simulink model "npc_controller"  (R2022a)
settings: Solver=FixedStepDiscrete  StartTime=0.0  StopTime=20  RelTol=1e-3  EnableMultiTasking=on
values from neighbouring files (symbols this model uses):
  Tsw = 1.5E-5    [param.sldd]
undefined symbols (not defined in the file or in its folder): CAN_O_INT, CANA_BASE, Down, GPTRIP1SEL, GPTRIP2SEL, GPTRIP3SEL, TZ1, TZ2, TZ3, Up
libraries: simulink x153, hdlsllib x90, c2802xlib x34, c2837xDlib x18, c280xlib x12, canmsglib x9, c2838xlib x8, idelinklib_common x3, c2806xlib x2, slpidlib x2, c28004xlib x2, c281xlib x2
(part 11 of 45)

== system npc_controller/CONTROL/SVPWM/SVPWM2/detSeq ==
  subsector : Inport  OutDataTypeStr=double  PortDimensions=1
  f : TriggerPort  TriggerType=function-call  VariantControl=(inherit)
      settings: CopyFcn=Stateflow.SLINSF.SimulinkMan.removeBlockPreDeleteFcn  PreDeleteFcn=Stateflow.SLINSF.SimulinkMan.unsafePredeleteFcn
  Cast To Double : DataTypeConversion  OutDataTypeStr=double  SaturateOnIntegerOverflow=off  RndMeth=Floor
  Cast To Double1 : DataTypeConversion  OutDataTypeStr=double  SaturateOnIntegerOverflow=off  RndMeth=Floor
  Cast To Double2 : DataTypeConversion  OutDataTypeStr=double  SaturateOnIntegerOverflow=off  RndMeth=Floor
  Constant{,5,7..8,12,17} (6 alike) : Constant  Value=[0 1 1 1]
  Constant1 : Constant  Value=[0 1 0 1]
  Constant{2..3,10..11,14..15} (6 alike) : Constant  Value=[0 0 0 1]
  Constant13 : Constant  Value=[0 1 0 1]
  Constant16 : Constant  Value=[0 0 1 1]
  Constant18 : Constant  Commented=on  Value=[1 1 0 0]
  Constant19 : Constant  Commented=on  Value=[1 0 0 0]
  Constant20 : Constant  Commented=on  Value=[1 1 1 0]
  Constant21 : Constant  Commented=on  Value=[1 1 1 0]
  Constant22 : Constant  Commented=on  Value=[1 1 0 0]
  Constant23 : Constant  Commented=on  Value=[1 0 0 0]
  Constant24 : Constant  Commented=on  Value=[1 0 0 0]
  Constant25 : Constant  Commented=on  Value=[1 1 1 0]
  Constant26 : Constant  Commented=on  Value=[1 1 0 0]
  Constant4 : Constant  Value=[0 0 1 1]
  Constant6 : Constant  Value=[0 0 1 1]
  Constant9 : Constant  Value=[0 1 0 1]
  Multiport Switch : MultiPortSwitch  Inputs=6  DataPortForDefault=Additional data port  SaturateOnIntegerOverflow=off  InputSameDT=off
  Multiport Switch1 : MultiPortSwitch  Inputs=6  DataPortForDefault=Additional data port  SaturateOnIntegerOverflow=off  InputSameDT=off
  Multiport Switch2 : MultiPortSwitch  Inputs=6  DataPortForDefault=Additional data port  SaturateOnIntegerOverflow=off  InputSameDT=off
  r_seq : Outport
  s_seq : Outport  Port=2
  t_seq : Outport  Port=3
  wires:
  Multiport Switch2/1 -> Cast To Double2/1
  Constant15/1 -> Multiport Switch2/3
  Constant16/1 -> Multiport Switch2/4
  Constant17/1 -> Multiport Switch2/5
  Constant12/1 -> Multiport Switch2/6
  Constant13/1 -> Multiport Switch2/7
  Constant14/1 -> Multiport Switch2/2
  [subsector] -> Multiport Switch2/1
  Multiport Switch1/1 -> Cast To Double1/1
  [subsector] -> Multiport Switch1/1
  Constant6/1 -> Multiport Switch1/2
  Constant11/1 -> Multiport Switch1/7
  Constant10/1 -> Multiport Switch1/6
  Constant9/1 -> Multiport Switch1/5
  Constant8/1 -> Multiport Switch1/4
  Constant7/1 -> Multiport Switch1/3
  Constant1/1 -> Multiport Switch/3
  Constant2/1 -> Multiport Switch/4
  Constant3/1 -> Multiport Switch/5
  Constant4/1 -> Multiport Switch/6
  Constant5/1 -> Multiport Switch/7
  Constant/1 -> Multiport Switch/2
  [subsector] -> Multiport Switch/1
  subsector/1 -> [subsector]
  Multiport Switch/1 -> Cast To Double/1
  Cast To Double/1 -> r_seq/1
  Cast To Double1/1 -> s_seq/1
  Cast To Double2/1 -> t_seq/1

== system npc_controller/CONTROL/SVPWM/SVPWM_with_bal/calcCmp ==
  r_seq : Inport  OutDataTypeStr=double  PortDimensions=4
  s_seq : Inport  Port=2  OutDataTypeStr=double  PortDimensions=4
  t_seq : Inport  Port=3  OutDataTypeStr=double  PortDimensions=4
  Tx : Inport  Port=4  OutDataTypeStr=double  PortDimensions=1
  Ty : Inport  Port=5  OutDataTypeStr=double  PortDimensions=1
  Tz : Inport  Port=6  OutDataTypeStr=double  PortDimensions=1
  f : TriggerPort  TriggerType=function-call  VariantControl=(inherit)
      settings: CopyFcn=Stateflow.SLINSF.SimulinkMan.removeBlockPreDeleteFcn  PreDeleteFcn=Stateflow.SLINSF.SimulinkMan.unsafePredeleteFcn
  Add : Sum  Inputs=++++
  Add1 : Sum  Inputs=++++
  Add2 : Sum  Inputs=++++
  Demux : Demux
  Demux1 : Demux
  Demux2 : Demux
  Gain{,2,5,7,10,12} (6 alike) : Gain  Gain=0.5
  Gain1 : Gain  Gain=1/15e-6
  Gain11 : Gain  Gain=1/15e-6
  Gain6 : Gain  Gain=1/15e-6
  Product{,1..11} (12 alike) : Product
  cmp_r : Outport
  cmp_s : Outport  Port=2
  cmp_t : Outport  Port=3
  wires:
  r_seq/1 -> [r_seq]
  Ty/1 -> [Ty]
  Tx/1 -> [Tx]
  Tz/1 -> [Tz]
  [r_seq] -> Demux/1
  [Tz] -> Gain/1
  Add/1 -> Gain1/1
  Gain1/1 -> cmp_r/1
  [Tz] -> Gain2/1
  Product/1 -> Add/1
  Gain/1 -> Product/2
  Demux/1 -> Product/1
  Product1/1 -> Add/2
  Product2/1 -> Add/3
  Product3/1 -> Add/4
  Demux/2 -> Product1/1
  Demux/3 -> Product2/1
  Demux/4 -> Product3/1
  [Tx] -> Product1/2
  [Ty] -> Product2/2
  Gain2/1 -> Product3/2
  Gain7/1 -> Product7/2
  [Ty] -> Product6/2
  [Tx] -> Product5/2
  Demux1/4 -> Product7/1
  Demux1/3 -> Product6/1
  Demux1/2 -> Product5/1
  Product7/1 -> Add1/4
  Product6/1 -> Add1/3
  Product5/1 -> Add1/2
  Demux1/1 -> Product4/1
  Gain5/1 -> Product4/2
  Product4/1 -> Add1/1
  [Tz] -> Gain7/1
  Add1/1 -> Gain6/1
  [Tz] -> Gain5/1
  [s_seq] -> Demux1/1
  Gain6/1 -> cmp_s/1
  [t_seq] -> Demux2/1
  [Tz] -> Gain10/1
  Add2/1 -> Gain11/1
  [Tz] -> Gain12/1
  Product8/1 -> Add2/1
  Gain10/1 -> Product8/2
  Demux2/1 -> Product8/1
  Product9/1 -> Add2/2
  Product10/1 -> Add2/3
  Product11/1 -> Add2/4
  Demux2/2 -> Product9/1
  Demux2/3 -> Product10/1
  Demux2/4 -> Product11/1
  [Tx] -> Product9/2
  [Ty] -> Product10/2
  Gain12/1 -> Product11/2
  Gain11/1 -> cmp_t/1
  t_seq/1 -> [t_seq]
  s_seq/1 -> [s_seq]

== system npc_controller/CONTROL/SVPWM/SVPWM_with_bal/calcCmpWithBal ==
  r_seq : Inport  OutDataTypeStr=double  PortDimensions=4
  s_seq : Inport  Port=2  OutDataTypeStr=double  PortDimensions=4
  t_seq : Inport  Port=3  OutDataTypeStr=double  PortDimensions=4
  Tx : Inport  Port=4  OutDataTypeStr=double  PortDimensions=1
  Ty : Inport  Port=5  OutDataTypeStr=double  PortDimensions=1
  Tz : Inport  Port=6  OutDataTypeStr=double  PortDimensions=1
  f : TriggerPort  TriggerType=function-call  VariantControl=(inherit)
      settings: CopyFcn=Stateflow.SLINSF.SimulinkMan.removeBlockPreDeleteFcn  PreDeleteFcn=Stateflow.SLINSF.SimulinkMan.unsafePredeleteFcn
  Add : Sum  Inputs=++++
  Add1 : Sum  Inputs=++++
  Add2 : Sum  Inputs=++++
  Demux : Demux
  Demux1 : Demux
  Demux2 : Demux
  Gain{,2,5,7,10,12} (6 alike) : Gain  Gain=0.5
  Gain1 : Gain  Gain=1/15e-6
  Gain11 : Gain  Gain=1/15e-6
  Gain6 : Gain  Gain=1/15e-6
  Product{,1..11} (12 alike) : Product
  cmp_r : Outport
  cmp_s : Outport  Port=2
  cmp_t : Outport  Port=3
  wires:
  r_seq/1 -> [r_seq]
  Ty/1 -> [Ty]
  Tx/1 -> [Tx]
  Tz/1 -> [Tz]
  [r_seq] -> Demux/1
  [Tz] -> Gain/1
  Add/1 -> Gain1/1
  Gain1/1 -> cmp_r/1
  [Tz] -> Gain2/1
  Product/1 -> Add/1
  Gain/1 -> Product/2
  Demux/1 -> Product/1
  Product1/1 -> Add/2
  Product2/1 -> Add/3
  Product3/1 -> Add/4
  Demux/2 -> Product1/1
  Demux/3 -> Product2/1
  Demux/4 -> Product3/1
  [Tx] -> Product1/2
  [Ty] -> Product2/2
  Gain2/1 -> Product3/2
  Gain7/1 -> Product7/2
  [Ty] -> Product6/2
  [Tx] -> Product5/2
  Demux1/4 -> Product7/1
  Demux1/3 -> Product6/1
  Demux1/2 -> Product5/1
  Product7/1 -> Add1/4
  Product6/1 -> Add1/3
  Product5/1 -> Add1/2
  Demux1/1 -> Product4/1
  Gain5/1 -> Product4/2
  Product4/1 -> Add1/1
  [Tz] -> Gain7/1
  Add1/1 -> Gain6/1
  [Tz] -> Gain5/1
  [s_seq] -> Demux1/1
  Gain6/1 -> cmp_s/1
  [t_seq] -> Demux2/1
  [Tz] -> Gain10/1
  Add2/1 -> Gain11/1
  [Tz] -> Gain12/1
  Product8/1 -> Add2/1
  Gain10/1 -> Product8/2
  Demux2/1 -> Product8/1
  Product9/1 -> Add2/2
  Product10/1 -> Add2/3
  Product11/1 -> Add2/4
  Demux2/2 -> Product9/1
  Demux2/3 -> Product10/1
  Demux2/4 -> Product11/1
  [Tx] -> Product9/2
  [Ty] -> Product10/2
  Gain12/1 -> Product11/2
  Gain11/1 -> cmp_t/1
  t_seq/1 -> [t_seq]
  s_seq/1 -> [s_seq]

== system npc_controller/CONTROL/SVPWM/SVPWM_with_bal/calcDwellingTimes ==
  Tsw : Inport  OutDataTypeStr=double  PortDimensions=1
  vref_fict_mag_alpha : Inport  Port=2  OutDataTypeStr=double  PortDimensions=1
  vref_fict_mag_beta : Inport  Port=3  OutDataTypeStr=double  PortDimensions=1
  vx_fict_mag_alpha : Inport  Port=4  OutDataTypeStr=double  PortDimensions=1
  vx_fict_mag_beta : Inport  Port=5  OutDataTypeStr=double  PortDimensions=1
  vy_fict_mag_alpha : Inport  Port=6  OutDataTypeStr=double  PortDimensions=1
  vy_fict_mag_beta : Inport  Port=7  OutDataTypeStr=double  PortDimensions=1
  f : TriggerPort  TriggerType=function-call  VariantControl=(inherit)
      settings: CopyFcn=Stateflow.SLINSF.SimulinkMan.removeBlockPreDeleteFcn  PreDeleteFcn=Stateflow.SLINSF.SimulinkMan.unsafePredeleteFcn
  Add : Sum  Inputs=+-
  Add1 : Sum  Inputs=+--
  Cast To Single : DataTypeConversion  OutDataTypeStr=single  SaturateOnIntegerOverflow=off  RndMeth=Floor
  Cast To Single1 : DataTypeConversion  OutDataTypeStr=single  SaturateOnIntegerOverflow=off  RndMeth=Floor
  Cast To Single2 : DataTypeConversion  OutDataTypeStr=single  SaturateOnIntegerOverflow=off  RndMeth=Floor
  Display{,1..17} (18 alike) : Display
  Divide : Product  Inputs=**/
  Divide1 : Product  Inputs=*/
  Product{,1..5} (6 alike) : Product
  Subtract : Sum  Inputs=+-
  Subtract1 : Sum  Inputs=+-
  Tx : Outport
  Ty : Outport  Port=2
  Tz : Outport  Port=3
  wires:
  [vx_fict_mag_beta] -> Product2/1
  [vy_fict_mag_alpha] -> Product2/2
  [Tsw] -> Display17/1, Divide/1
  Cast To Single2/1 -> Tz/1
  Cast To Single1/1 -> Ty/1
  Cast To Single/1 -> Tx/1
  [Tsw] -> Add1/1
  [Tx] -> Add1/2
  [Ty] -> Add1/3
  [vy_fict_mag_alpha] -> Divide1/2
  Subtract1/1 -> Divide1/1
  Product5/1 -> Subtract1/2
  [Tx] -> Product5/2
  [vx_fict_mag_alpha] -> Product5/1
  [Tsw] -> Product4/2
  [vref_fict_mag_alpha] -> Product4/1
  Product4/1 -> Subtract1/1, Display/1
  Subtract/1 -> Display16/1, Divide/3
  Add/1 -> Display11/1, Divide/2
  Product3/1 -> Display14/1, Subtract/2
  Product2/1 -> Display15/1, Subtract/1
  Product1/1 -> Display13/1, Add/2
  Product/1 -> Display12/1, Add/1
  [vy_fict_mag_beta] -> Product3/2
  [vx_fict_mag_alpha] -> Product3/1
  [vy_fict_mag_beta] -> Product1/2
  [vref_fict_mag_alpha] -> Product1/1
  [vy_fict_mag_alpha] -> Product/2
  [vref_fict_mag_beta] -> Product/1
  vy_fict_mag_beta/1 -> [vy_fict_mag_beta], Display10/1
  vy_fict_mag_alpha/1 -> [vy_fict_mag_alpha], Display9/1
  vx_fict_mag_beta/1 -> [vx_fict_mag_beta], Display8/1
  vx_fict_mag_alpha/1 -> [vx_fict_mag_alpha], Display7/1
  vref_fict_mag_beta/1 -> [vref_fict_mag_beta], Display6/1
  vref_fict_mag_alpha/1 -> [vref_fict_mag_alpha], Display5/1
  Tsw/1 -> [Tsw], Display4/1
  Divide/1 -> [Tx], Display1/1, Cast To Single/1
  Divide1/1 -> Cast To Single1/1, [Ty], Display2/1
  Add1/1 -> Cast To Single2/1, Display3/1

== system npc_controller/CONTROL/SVPWM/SVPWM_with_bal/detSeq ==
  subsector : Inport  OutDataTypeStr=double  PortDimensions=1
  f : TriggerPort  TriggerType=function-call  VariantControl=(inherit)
      settings: CopyFcn=Stateflow.SLINSF.SimulinkMan.removeBlockPreDeleteFcn  PreDeleteFcn=Stateflow.SLINSF.SimulinkMan.unsafePredeleteFcn
  Cast To Double : DataTypeConversion  OutDataTypeStr=double  SaturateOnIntegerOverflow=off  RndMeth=Floor
  Cast To Double1 : DataTypeConversion  OutDataTypeStr=double  SaturateOnIntegerOverflow=off  RndMeth=Floor
  Cast To Double2 : DataTypeConversion  OutDataTypeStr=double  SaturateOnIntegerOverflow=off  RndMeth=Floor
  Constant : Constant  Value=[0 1 1 1]
  Constant1 : Constant  Value=[1 1 0 0]
  Constant10 : Constant  Value=[0 0 0 1]
  Constant11 : Constant  Value=[1 0 0 0]
  Constant12 : Constant  Value=[0 1 1 1]
  Constant13 : Constant  Value=[1 1 0 0]
  Constant14 : Constant  Value=[0 0 0 1]
  Constant15 : Constant  Value=[1 0 0 0]
  Constant16 : Constant  Value=[0 0 1 1]
  Constant17 : Constant  Value=[1 1 1 0]
  Constant2 : Constant  Value=[0 0 0 1]
  Constant3 : Constant  Value=[1 0 0 0]
  Constant4 : Constant  Value=[0 0 1 1]
  Constant5 : Constant  Value=[1 1 1 0]
  Constant6 : Constant  Value=[0 0 1 1]
  Constant7 : Constant  Value=[1 1 1 0]
  Constant8 : Constant  Value=[0 1 1 1]
  Constant9 : Constant  Value=[1 1 0 0]
  Multiport Switch : MultiPortSwitch  Inputs=6  DataPortForDefault=Additional data port  SaturateOnIntegerOverflow=off  InputSameDT=off
  Multiport Switch1 : MultiPortSwitch  Inputs=6  DataPortForDefault=Additional data port  SaturateOnIntegerOverflow=off  InputSameDT=off
  Multiport Switch2 : MultiPortSwitch  Inputs=6  DataPortForDefault=Additional data port  SaturateOnIntegerOverflow=off  InputSameDT=off
  r_seq : Outport
  s_seq : Outport  Port=2
  t_seq : Outport  Port=3
  wires:
  Cast To Double2/1 -> t_seq/1
  Cast To Double1/1 -> s_seq/1
  Cast To Double/1 -> r_seq/1
  Multiport Switch/1 -> Cast To Double/1
  subsector/1 -> [subsector]
  [subsector] -> Multiport Switch/1
  Constant/1 -> Multiport Switch/2
  Constant5/1 -> Multiport Switch/7
  Constant4/1 -> Multiport Switch/6
  Constant3/1 -> Multiport Switch/5
  Constant2/1 -> Multiport Switch/4
  Constant1/1 -> Multiport Switch/3
  Constant7/1 -> Multiport Switch1/3
  Constant8/1 -> Multiport Switch1/4
  Constant9/1 -> Multiport Switch1/5
  Constant10/1 -> Multiport Switch1/6
  Constant11/1 -> Multiport Switch1/7
  Constant6/1 -> Multiport Switch1/2
  [subsector] -> Multiport Switch1/1
  Multiport Switch1/1 -> Cast To Double1/1
  [subsector] -> Multiport Switch2/1
  Constant14/1 -> Multiport Switch2/2
  Constant13/1 -> Multiport Switch2/7
  Constant12/1 -> Multiport Switch2/6
  Constant17/1 -> Multiport Switch2/5
  Constant16/1 -> Multiport Switch2/4
  Constant15/1 -> Multiport Switch2/3
  Multiport Switch2/1 -> Cast To Double2/1

== system npc_controller/CONTROL/SVPWM/SVPWM_with_bal/detSeqFixedSmallVector ==
  subsector : Inport  OutDataTypeStr=double  PortDimensions=1
  f : TriggerPort  TriggerType=function-call  VariantControl=(inherit)
      settings: CopyFcn=Stateflow.SLINSF.SimulinkMan.removeBlockPreDeleteFcn  PreDeleteFcn=Stateflow.SLINSF.SimulinkMan.unsafePredeleteFcn
  Cast To Double : DataTypeConversion  OutDataTypeStr=double  SaturateOnIntegerOverflow=off  RndMeth=Floor
  Cast To Double1 : DataTypeConversion  OutDataTypeStr=double  SaturateOnIntegerOverflow=off  RndMeth=Floor
  Cast To Double2 : DataTypeConversion  OutDataTypeStr=double  SaturateOnIntegerOverflow=off  RndMeth=Floor
  Constant{,7..8,12,17} (5 alike) : Constant  Value=[0 1 1 1]
  Constant1 : Constant  Value=[1 1 0 0]
  Constant{2,10..11,14..15} (5 alike) : Constant  Value=[0 0 0 1]
  Constant13 : Constant  Value=[0 1 0 1]
  Constant16 : Constant  Value=[0 0 1 1]
  Constant18 : Constant  Commented=on  Value=[1 1 0 0]
  Constant19 : Constant  Commented=on  Value=[1 0 0 0]
  Constant20 : Constant  Commented=on  Value=[1 1 1 0]
  Constant21 : Constant  Commented=on  Value=[1 1 1 0]
  Constant22 : Constant  Commented=on  Value=[1 1 0 0]
  Constant23 : Constant  Commented=on  Value=[1 0 0 0]
  Constant24 : Constant  Commented=on  Value=[1 0 0 0]
  Constant25 : Constant  Commented=on  Value=[1 1 1 0]
  Constant26 : Constant  Commented=on  Value=[1 1 0 0]
  Constant3 : Constant  Value=[1 0 0 0]
  Constant4 : Constant  Value=[0 0 1 1]
  Constant5 : Constant  Value=[1 1 1 0]
  Constant6 : Constant  Value=[0 0 1 1]
  Constant9 : Constant  Value=[0 1 0 1]
  Multiport Switch : MultiPortSwitch  Inputs=6  DataPortForDefault=Additional data port  SaturateOnIntegerOverflow=off  InputSameDT=off
  Multiport Switch1 : MultiPortSwitch  Inputs=6  DataPortForDefault=Additional data port  SaturateOnIntegerOverflow=off  InputSameDT=off
  Multiport Switch2 : MultiPortSwitch  Inputs=6  DataPortForDefault=Additional data port  SaturateOnIntegerOverflow=off  InputSameDT=off
  r_seq : Outport
  s_seq : Outport  Port=2
  t_seq : Outport  Port=3
  wires:
  Cast To Double2/1 -> t_seq/1
  Cast To Double1/1 -> s_seq/1
  Cast To Double/1 -> r_seq/1
  Multiport Switch/1 -> Cast To Double/1
  subsector/1 -> [subsector]
  [subsector] -> Multiport Switch/1
  Constant/1 -> Multiport Switch/2
  Constant5/1 -> Multiport Switch/7
  Constant4/1 -> Multiport Switch/6
  Constant3/1 -> Multiport Switch/5
  Constant2/1 -> Multiport Switch/4
  Constant1/1 -> Multiport Switch/3
  Constant7/1 -> Multiport Switch1/3
  Constant8/1 -> Multiport Switch1/4
  Constant9/1 -> Multiport Switch1/5
  Constant10/1 -> Multiport Switch1/6
  Constant11/1 -> Multiport Switch1/7
  Constant6/1 -> Multiport Switch1/2
  [subsector] -> Multiport Switch1/1
  Multiport Switch1/1 -> Cast To Double1/1
  [subsector] -> Multiport Switch2/1
  Constant14/1 -> Multiport Switch2/2
  Constant13/1 -> Multiport Switch2/7
  Constant12/1 -> Multiport Switch2/6
  Constant17/1 -> Multiport Switch2/5
  Constant16/1 -> Multiport Switch2/4
  Constant15/1 -> Multiport Switch2/3
  Multiport Switch2/1 -> Cast To Double2/1

== system npc_controller/CONTROL/SVPWM/Subsystem ==
  Trigger : TriggerPort  TriggerType=function-call  VariantControl=Variant  PortDimensions=1
  Constant16 : Constant
  Out1 : Outport
  wires:
  Constant16/1 -> Out1/1

== system npc_controller/CONTROL/SVPWM/Subsystem1 ==
  note: interacting PID
  error : Inport
  disable : Inport  Port=2
  Constant : Constant  Value=18.57
  Constant1 : Constant  Value=-34.95
  Constant2 : Constant  Value=470
  Constant3 : Constant  Value=-470
  Constant4 : Constant  Value=16.46
  Constant5 : Constant  Value=-1.246
  Constant6 : Constant  Value=0.2457
  Delay{1..4} (4 alike) : Delay  DelayLength=1  InitialCondition=0  ExternalReset=Level
      settings: InputPortMap=u0,r5
  Product{1..5} (5 alike) : Product
  Saturation Dynamic1 : simulink/Discontinuities/Saturation Dynamic  OutMin=[]  OutMax=[]  OutDataTypeStr=double  OutputDataTypeScalingMode=double  OutDataType=fixdt(1, 16)  OutScaling=2^-10  DoSatur=off
  Scope : Scope  NumInputPorts=4
  Sum : Sum  Inputs=|+++--
  pi : Outport
  wires:
  [error] -> Scope/1  "error"
  [kP_term] -> Scope/2  "kP_term"
  [kI_term] -> Scope/3  "kI_term"
  [pi] -> Scope/4  "PI"
  [a0] -> Product3/2
  Sum/1 -> Saturation Dynamic1/2
  [integ_min] -> Saturation Dynamic1/3
  [integ_max] -> Saturation Dynamic1/1
  Constant2/1 -> [integ_max]
  Constant3/1 -> [integ_min]
  Constant1/1 -> [a1]
  error/1 -> [error]
  [a1] -> Product2/2
  Constant/1 -> [a0]
  [error] -> Delay2/1, Product3/1
  Delay2/1 -> Product2/1, Delay3/1
  Saturation Dynamic1/1 -> pi/1, Delay1/1, [pi]
  Delay3/1 -> Product1/1
  [a2] -> Product1/2
  Product3/1 -> Sum/1
  Product2/1 -> Sum/2
  Product1/1 -> Sum/3
  Delay1/1 -> Product4/2, Delay4/1
  [b1] -> Product4/1
  Delay4/1 -> Product5/2
  Product5/1 -> Sum/5
  Product4/1 -> Sum/4
  [b2] -> Product5/1
  Constant5/1 -> [b1]
  Constant4/1 -> [a2]
  Constant6/1 -> [b2]
  disable/1 -> Delay4/2, Delay1/2, Delay3/2, Delay2/2

== system npc_controller/CONTROL/SVPWM/Subsystem2 ==
  note: Parallel PI
  error : Inport
  Constant : Constant  Value=0.3055
  Constant1 : Constant  Value=-0.3052
  Constant2 : Constant  Value=50
  Constant3 : Constant  Value=-50
  Constant4 : Constant  Commented=on  Value=36
  Constant5 : Constant  Commented=on  Value=-36
  Constant6 : Constant  Commented=on  Value=0.611
  Constant7 : Constant  Commented=on  Value=-0.6105
  Delay1 : Delay  DelayLength=1  InitialCondition=22
  Delay2 : Delay  DelayLength=1  InitialCondition=0
  Product2 : Product
  Product3 : Product
  Saturation Dynamic1 : simulink/Discontinuities/Saturation Dynamic  OutMin=[]  OutMax=[]  OutDataTypeStr=double  OutputDataTypeScalingMode=double  OutDataType=fixdt(1, 16)  OutScaling=2^-10  DoSatur=off
  Scope : Scope  NumInputPorts=4
  Sum : Sum  Inputs=|++
  Sum3 : Sum  Inputs=|++
  pi : Outport
  wires:
  Saturation Dynamic1/1 -> [pi], Delay1/1, pi/1
  Delay2/1 -> Product2/1
  [error] -> Delay2/1
  Sum3/1 -> Sum/2, [kI_term]
  Delay1/1 -> Sum3/2
  Constant/1 -> [kp]
  [ki] -> Product2/2
  error/1 -> [error]
  Constant1/1 -> [ki]
  [error] -> Product3/1
  Product3/1 -> [kP_term], Sum/1
  Product2/1 -> Sum3/1
  Constant3/1 -> [integ_min]
  Constant2/1 -> [integ_max]
  [integ_max] -> Saturation Dynamic1/1
  [integ_min] -> Saturation Dynamic1/3
  Sum/1 -> Saturation Dynamic1/2
  [kp] -> Product3/2
  [pi] -> Scope/4  "PI"
  [kI_term] -> Scope/3  "kI_term"
  [kP_term] -> Scope/2  "kP_term"
  [error] -> Scope/1  "error"

== system npc_controller/CONTROL/SVPWM/Subsystem4 ==
  note: interacting PID
  error : Inport
  disable : Inport  Port=2
  Constant : Constant  Value=18.57
  Constant1 : Constant  Value=-34.95
  Constant2 : Constant  Value=470
  Constant3 : Constant  Value=-470
  Constant4 : Constant  Value=16.46
  Constant5 : Constant  Value=-1.246
  Constant6 : Constant  Value=0.2457
  Delay{1..4} (4 alike) : Delay  DelayLength=1  InitialCondition=0  ExternalReset=Level
      settings: InputPortMap=u0,r5
  Product{1..5} (5 alike) : Product
  Saturation Dynamic1 : simulink/Discontinuities/Saturation Dynamic  OutMin=[]  OutMax=[]  OutDataTypeStr=double  OutputDataTypeScalingMode=double  OutDataType=fixdt(1, 16)  OutScaling=2^-10  DoSatur=off
  Scope : Scope  NumInputPorts=4
  Sum : Sum  Inputs=|+++--
  pi : Outport
  wires:
  disable/1 -> Delay2/2, Delay3/2, Delay1/2, Delay4/2
  Constant6/1 -> [b2]
  Constant4/1 -> [a2]
  Constant5/1 -> [b1]
  [b2] -> Product5/1
  Product4/1 -> Sum/4
  Product5/1 -> Sum/5
  Delay4/1 -> Product5/2
  [b1] -> Product4/1
  Delay1/1 -> Delay4/1, Product4/2
  Product1/1 -> Sum/3
  Product2/1 -> Sum/2
  Product3/1 -> Sum/1
  [a2] -> Product1/2
  Delay3/1 -> Product1/1
  Saturation Dynamic1/1 -> [pi], Delay1/1, pi/1
  Delay2/1 -> Delay3/1, Product2/1
  [error] -> Product3/1, Delay2/1
  Constant/1 -> [a0]
  [a1] -> Product2/2
  error/1 -> [error]
  Constant1/1 -> [a1]
  Constant3/1 -> [integ_min]
  Constant2/1 -> [integ_max]
  [integ_max] -> Saturation Dynamic1/1
  [integ_min] -> Saturation Dynamic1/3
  Sum/1 -> Saturation Dynamic1/2
  [a0] -> Product3/2
  [pi] -> Scope/4  "PI"
  [kI_term] -> Scope/3  "kI_term"
  [kP_term] -> Scope/2  "kP_term"
  [error] -> Scope/1  "error"

== system npc_controller/CONTROL/SVPWM/Subsystem5 ==
  note: Parallel PI
  error : Inport
  Constant : Constant  Value=0.611e-1
  Constant1 : Constant  Value=-0.6105e-1
  Constant2 : Constant  Value=0.8
  Constant3 : Constant  Value=0.2
  Constant4 : Constant  Commented=on  Value=36
  Constant5 : Constant  Commented=on  Value=-36
  Constant6 : Constant  Commented=on  Value=0.611e-1
  Constant7 : Constant  Commented=on  Value=-0.6105e-1
  Delay1 : Delay  DelayLength=1  InitialCondition=22
  Delay2 : Delay  DelayLength=1  InitialCondition=0
  Product2 : Product
  Product3 : Product
  Saturation Dynamic1 : simulink/Discontinuities/Saturation Dynamic  OutMin=[]  OutMax=[]  OutDataTypeStr=double  OutputDataTypeScalingMode=double  OutDataType=fixdt(1, 16)  OutScaling=2^-10  DoSatur=off
  Scope : Scope  NumInputPorts=4
  Sum : Sum  Inputs=|++
  Sum3 : Sum  Inputs=|++
  pi : Outport
  wires:
  Saturation Dynamic1/1 -> [pi], Delay1/1, pi/1
  Delay2/1 -> Product2/1
  [error] -> Delay2/1
  Sum3/1 -> Sum/2, [kI_term]
  Delay1/1 -> Sum3/2
  Constant/1 -> [kp]
  [ki] -> Product2/2
  error/1 -> [error]
  Constant1/1 -> [ki]
  [error] -> Product3/1
  Product3/1 -> [kP_term], Sum/1
  Product2/1 -> Sum3/1
  Constant3/1 -> [integ_min]
  Constant2/1 -> [integ_max]
  [integ_max] -> Saturation Dynamic1/1
  [integ_min] -> Saturation Dynamic1/3
  Sum/1 -> Saturation Dynamic1/2
  [kp] -> Product3/2
  [pi] -> Scope/4  "PI"
  [kI_term] -> Scope/3  "kI_term"
  [kP_term] -> Scope/2  "kP_term"
  [error] -> Scope/1  "error"

== system npc_controller/CONTROL/SVPWM/Subsystem6 ==
  note: Parallel PI
  error : Inport
  Constant : Constant  Value=1.407
  Constant1 : Constant  Value=-1.387
  Constant2 : Constant  Value=470
  Constant3 : Constant  Value=-470
  Constant4 : Constant  Commented=on  Value=470
  Constant5 : Constant  Commented=on  Value=-470
  Constant6 : Constant  Commented=on  Value=0.7034
  Constant7 : Constant  Commented=on  Value=-0.6871
  Delay1 : Delay  DelayLength=1  InitialCondition=0
  Delay2 : Delay  DelayLength=1  InitialCondition=0
  Product2 : Product
  Product3 : Product
  Saturation Dynamic1 : simulink/Discontinuities/Saturation Dynamic  OutMin=[]  OutMax=[]  OutDataTypeStr=double  OutputDataTypeScalingMode=double  OutDataType=fixdt(1, 16)  OutScaling=2^-10  DoSatur=off
  Scope : Scope  NumInputPorts=4
  Sum : Sum  Inputs=|++
  Sum3 : Sum  Inputs=|++
  pi : Outport
  wires:
  [error] -> Scope/1  "error"
  [kP_term] -> Scope/2  "kP_term"
  [kI_term] -> Scope/3  "kI_term"
  [pi] -> Scope/4  "PI"
  [kp] -> Product3/2
  Sum/1 -> Saturation Dynamic1/2
  [integ_min] -> Saturation Dynamic1/3
  [integ_max] -> Saturation Dynamic1/1
  Constant2/1 -> [integ_max]
  Constant3/1 -> [integ_min]
  Product2/1 -> Sum3/1
  Product3/1 -> Sum/1, [kP_term]
  [error] -> Product3/1
  Constant1/1 -> [ki]
  error/1 -> [error]
  [ki] -> Product2/2
  Constant/1 -> [kp]
  Delay1/1 -> Sum3/2
  Sum3/1 -> [kI_term], Sum/2
  [error] -> Delay2/1
  Delay2/1 -> Product2/1
  Saturation Dynamic1/1 -> pi/1, Delay1/1, [pi]

== system npc_controller/CONTROL/SVPWM/Subsystem7 ==
  note: Parallel PI
  error : Inport
  Constant : Constant  Value=1.407
  Constant1 : Constant  Value=-1.387
  Constant2 : Constant  Value=470
  Constant3 : Constant  Value=-470
  Constant4 : Constant  Commented=on  Value=470
  Constant5 : Constant  Commented=on  Value=-470
  Constant6 : Constant  Commented=on  Value=0.7034
  Constant7 : Constant  Commented=on  Value=-0.6871
  Delay1 : Delay  DelayLength=1  InitialCondition=0
  Delay2 : Delay  DelayLength=1  InitialCondition=0
  Product2 : Product
  Product3 : Product
  Saturation Dynamic1 : simulink/Discontinuities/Saturation Dynamic  OutMin=[]  OutMax=[]  OutDataTypeStr=double  OutputDataTypeScalingMode=double  OutDataType=fixdt(1, 16)  OutScaling=2^-10  DoSatur=off
  Scope : Scope  NumInputPorts=4
  Sum : Sum  Inputs=|++
  Sum3 : Sum  Inputs=|++
  pi : Outport
  wires:
  [error] -> Scope/1  "error"
  [kP_term] -> Scope/2  "kP_term"
  [kI_term] -> Scope/3  "kI_term"
  [pi] -> Scope/4  "PI"
  [kp] -> Product3/2
  Sum/1 -> Saturation Dynamic1/2
  [integ_min] -> Saturation Dynamic1/3
  [integ_max] -> Saturation Dynamic1/1
  Constant2/1 -> [integ_max]
  Constant3/1 -> [integ_min]
  Product2/1 -> Sum3/1
  Product3/1 -> Sum/1, [kP_term]
  [error] -> Product3/1
  Constant1/1 -> [ki]
  error/1 -> [error]
  [ki] -> Product2/2
  Constant/1 -> [kp]
  Delay1/1 -> Sum3/2
  Sum3/1 -> [kI_term], Sum/2
  [error] -> Delay2/1
  Delay2/1 -> Product2/1
  Saturation Dynamic1/1 -> pi/1, Delay1/1, [pi]

== system npc_controller/CONTROL/SVPWM/abc to dq ==
  note: wt
  note: wt
  note: wt
  note: wt
  note: wt
  note: wt
  abc : Inport
  wt : Inport  Port=2
  (wt+120) : Sum  Inputs=|++
  (wt-120) : Sum  Inputs=|+-
  2pi_3 : Constant  Value=2*pi/3
  Add2 : Sum  Inputs=+++
  Add3 : Sum  Inputs=+++
  Cos : Trigonometry
  Cos1 : Trigonometry
  Cos2 : Trigonometry
  Cos3 : Trigonometry  Operator=cos
  Cos4 : Trigonometry  Operator=cos
  Cos5 : Trigonometry  Operator=cos
  Demux : Demux  Outputs=3
  Mux : Mux  Inputs=3
  Product{2..7} (6 alike) : Product
  d1 : Gain  Gain=2/3
  q1 : Gain  Gain=2/3
  wt+120 : Sum  Inputs=|++
  wt-120 : Sum  Inputs=|+-
  dq0 : Outport
  wires:
  Mux/1 -> dq0/1
  abc/1 -> Demux/1
  2pi_3/1 -> [ph]
  q1/1 -> Mux/2
  [c] -> Product7/1
  Add3/1 -> q1/1
  [c] -> Product4/1
  wt-120/1 -> Cos1/1
  Demux/2 -> [b]
  [ph] -> wt-120/2
  Cos2/1 -> Product4/2
  wt+120/1 -> Cos2/1
  Cos5/1 -> Product7/2
  [ph] -> wt+120/2
  d1/1 -> Mux/1
  [b] -> Product3/1
  Product5/1 -> Add3/1
  Cos4/1 -> Product6/2
  [b] -> Product6/1
  (wt-120)/1 -> Cos4/1
  [ph] -> (wt-120)/2
  Demux/3 -> [c]
  Product6/1 -> Add3/2
  Product2/1 -> Add2/1
  (wt+120)/1 -> Cos5/1
  Product4/1 -> Add2/3
  Demux/1 -> [a]
  Product7/1 -> Add3/3
  [ph] -> (wt+120)/2
  Add2/1 -> d1/1
  wt/1 -> Cos3/1, (wt-120)/1, (wt+120)/1, wt+120/1, Cos/1, wt-120/1
  Product3/1 -> Add2/2
  [a] -> Product2/1
  Cos1/1 -> Product3/2
  Cos3/1 -> Product5/2
  Cos/1 -> Product2/2
  [a] -> Product5/1

== system npc_controller/CONTROL/SVPWM/abc to dq1 ==
  note: wt
  note: wt
  note: wt
  note: wt
  note: wt
  note: wt
  abc : Inport
  wt : Inport  Port=2
  (wt+120) : Sum  Inputs=|++
  (wt-120) : Sum  Inputs=|+-
  2pi_3 : Constant  Value=2*pi/3
  Add2 : Sum  Inputs=+++
  Add3 : Sum  Inputs=+++
  Cos : Trigonometry
  Cos1 : Trigonometry
  Cos2 : Trigonometry
  Cos3 : Trigonometry  Operator=cos
  Cos4 : Trigonometry  Operator=cos
  Cos5 : Trigonometry  Operator=cos
  Demux : Demux  Outputs=3
  Mux : Mux  Inputs=3
  Product{2..7} (6 alike) : Product
  d1 : Gain  Gain=2/3
  q1 : Gain  Gain=2/3
  wt+120 : Sum  Inputs=|++
  wt-120 : Sum  Inputs=|+-
  dq0 : Outport
  wires:
  [a] -> Product5/1
  Cos/1 -> Product2/2
  Cos3/1 -> Product5/2
  Cos1/1 -> Product3/2
  [a] -> Product2/1
  Product3/1 -> Add2/2
  wt/1 -> wt-120/1, Cos/1, wt+120/1, (wt+120)/1, (wt-120)/1, Cos3/1
  Add2/1 -> d1/1
  [ph] -> (wt+120)/2
  Product7/1 -> Add3/3
  Demux/1 -> [a]
  Product4/1 -> Add2/3
  (wt+120)/1 -> Cos5/1
  Product2/1 -> Add2/1
  Product6/1 -> Add3/2
  Demux/3 -> [c]
  [ph] -> (wt-120)/2
  (wt-120)/1 -> Cos4/1
  [b] -> Product6/1
  Cos4/1 -> Product6/2
  Product5/1 -> Add3/1
  [b] -> Product3/1
  d1/1 -> Mux/1
  [ph] -> wt+120/2
  Cos5/1 -> Product7/2
  wt+120/1 -> Cos2/1
  Cos2/1 -> Product4/2
  [ph] -> wt-120/2
  Demux/2 -> [b]
  wt-120/1 -> Cos1/1
  [c] -> Product4/1
  Add3/1 -> q1/1
  [c] -> Product7/1
  q1/1 -> Mux/2
  2pi_3/1 -> [ph]
  abc/1 -> Demux/1
  Mux/1 -> dq0/1

== system npc_controller/CONTROL/SVPWM/dq to abc2 ==
  note: wt
  note: wt
  note: wt
  note: wt
  dq : Inport
  wt : Inport  Port=2
  (wt-120) : Sum  Inputs=|+-
  2pi_3 : Constant  Value=2*pi/3
  Cos : Trigonometry
  Cos1 : Trigonometry  Operator=cos
  Cos2 : Trigonometry
  Cos3 : Trigonometry  Operator=cos
  Cos4 : Trigonometry
  Cos5 : Trigonometry  Operator=cos
  Demux : Demux  Outputs=3
  Mux : Mux  Inputs=3
  Product{1..4,6..7} (6 alike) : Product
  a1 : Sum
  b1 : Sum
  c1 : Sum
  wt+120 : Sum  Inputs=|++
  abc : Outport
  wires:
  Demux/2 -> [q]
  Demux/1 -> [d]
  dq/1 -> Demux/1
  c1/1 -> Mux/3
  b1/1 -> Mux/2
  a1/1 -> Mux/1
  Mux/1 -> abc/1
  2pi_3/1 -> [ph]
  [q] -> Product7/1
  Cos5/1 -> Product7/2
  [q] -> Product3/1
  Cos4/1 -> Product6/2
  [d] -> Product6/1
  (wt-120)/1 -> Cos5/1, Cos4/1
  [ph] -> (wt-120)/2
  Product2/1 -> a1/1
  Product3/1 -> a1/2
  [d] -> Product2/1
  Cos1/1 -> Product3/2
  Cos/1 -> Product2/2
  Product6/1 -> b1/1
  Product7/1 -> b1/2
  Product4/1 -> c1/2
  Product1/1 -> c1/1
  wt/1 -> wt+120/1, (wt-120)/1, Cos1/1, Cos/1
  [ph] -> wt+120/2
  wt+120/1 -> Cos2/1, Cos3/1
  [d] -> Product1/1
  Cos2/1 -> Product1/2
  Cos3/1 -> Product4/2
  [q] -> Product4/1

== system npc_controller/IDLE_AND_TIMER/codegen/CAN_Task ==
  Trigger : TriggerPort  TriggerType=function-call  VariantControl=Variant  PortDimensions=1
  Function-Call Generator1 : simulink/Ports & Subsystems/Function-Call Generator  sample_time=-1  numberOfIterations=1  DisallowWideOutput=off
  Function-Call Split1 : FunctionCallSplit  NumOutputPorts=2
  Rx_Handler : Subsystem  TreatAsAtomicUnit=on
  Tx_Handler : Subsystem  TreatAsAtomicUnit=on
  wires:
  Function-Call Split1/1 -> Rx_Handler/Trigger
  Function-Call Generator1/1 -> Function-Call Split1/1
  Function-Call Split1/2 -> Tx_Handler/Trigger

== system npc_controller/IDLE_AND_TIMER/codegen/IDLE ==
  note: Note: GPIO6 J8.80
  note: Note: change to function call
  function : TriggerPort  TriggerType=function-call  VariantControl=Variant
  Function-Call Generator1 : simulink/Ports & Subsystems/Function-Call Generator  sample_time=-1  numberOfIterations=1  DisallowWideOutput=off
  Function-Call Split1 : FunctionCallSplit  NumOutputPorts=2
  Function-Call Split2 : FunctionCallSplit  NumOutputPorts=2
  Function-Call Split3 : FunctionCallSplit  NumOutputPorts=2
  GPIO6_HIGH : Subsystem  Commented=on
      settings: RTWSystemCode=Inline
  GPIO6_LOW : Subsystem  Commented=on
      settings: RTWSystemCode=Inline
  cnt_idle : Subsystem  TreatAsAtomicUnit=on
      settings: RTWSystemCode=Inline
  idle_task : Subsystem  TreatAsAtomicUnit=on
      settings: RTWSystemCode=Inline
  idle_task1 : Subsystem  Commented=on  TreatAsAtomicUnit=on
      settings: RTWSystemCode=Inline
  wires:
  Function-Call Split1/1 -> idle_task/Trigger
  Function-Call Split1/2 -> Function-Call Split2/1
  Function-Call Generator1/1 -> Function-Call Split3/1
  Function-Call Split3/1 -> GPIO6_HIGH/Trigger
  Function-Call Split3/2 -> Function-Call Split1/1
  Function-Call Split2/1 -> cnt_idle/Trigger
  Function-Call Split2/2 -> GPIO6_LOW/Trigger

== system npc_controller/IDLE_AND_TIMER/codegen/INITIALIZATION ==
  Function-Call Generator1 : simulink/Ports & Subsystems/Function-Call Generator  sample_time=-1  numberOfIterations=1  DisallowWideOutput=off
  Function-Call Split{1..3,5} (4 alike) : FunctionCallSplit  NumOutputPorts=2
  clb : Subsystem  Commented=on  TreatAsAtomicUnit=on
      settings: RTWSystemCode=Inline
  cmpss : Subsystem  TreatAsAtomicUnit=on
      settings: RTWSystemCode=Inline
  epwm : Subsystem  TreatAsAtomicUnit=on
      settings: RTWSystemCode=Inline
  epwm1 : Subsystem  Commented=on  TreatAsAtomicUnit=on
      settings: RTWSystemCode=Inline
  orps&relay : Subsystem  TreatAsAtomicUnit=on
      settings: RTWSystemCode=Inline
  outputxbar : Subsystem  Commented=on  TreatAsAtomicUnit=on
      settings: RTWSystemCode=Inline
  wires:
  Function-Call Generator1/1 -> Function-Call Split1/1
  Function-Call Split5/1 -> cmpss/Trigger
  Function-Call Split2/2 -> clb/Trigger
  Function-Call Split3/2 -> Function-Call Split5/1
  Function-Call Split2/1 -> outputxbar/Trigger
  Function-Call Split5/2 -> Function-Call Split2/1
  Function-Call Split3/1 -> orps&relay/Trigger
  Function-Call Split1/2 -> Function-Call Split3/1
  Function-Call Split1/1 -> epwm/Trigger

== system npc_controller/IDLE_AND_TIMER/codegen/TIMER_100MS ==
  note: Note: launchpad CANA, 32, 33
  note: Note:
      | Byte0 - func ID
      | Byte1 - MSB
      | Byte2 - LSB
  CAN Pack1 : canmsglib/CAN Pack  MsgList=(none)  MsgName=CAN Msg  MsgIDType=Standard (11-bit identifier)  MsgIdentifier=2  MsgLength=8  Remote=off  ApplyMinMax=off  BusOutput=off  SignalInfo={}
      settings: SourceProductBaseCode=ME,VN  DataFormat=raw data
  contstruct_can_msg : Subsystem
  eCAN Transmit : c280xlib/eCAN Transmit  chipFamily=C280x  useModule=eCAN_B  mailboxNo=1  messageID=bin2dec('111000111')  messageType=Standard (11-bit identifier)  enableBlockingMode=off  postInterrupt=off  interruptLine=0
      settings: SourceProductBaseCode=TIC2000
  get_func_id_data : Subsystem
  incr_cnt : Subsystem
  wires:
  CAN Pack1/1 -> eCAN Transmit/1
  contstruct_can_msg/1(can_msg) -> CAN Pack1/1
  get_func_id_data/2(data) -> contstruct_can_msg/2(data)
  get_func_id_data/1(func_id) -> contstruct_can_msg/1(func_id)

== system npc_controller/IDLE_AND_TIMER/codegen/TIMER_1MS ==
  note: 1) Add Subsystem or Model blocks as valid variant choices.
      | 2) You cannot connect blocks at this level. At simulation, connectivity is automatically
      | determined, based on the active variant and port name matching.
  codegen : Subsystem  VariantControl=sim_en==0
  sim : Subsystem  VariantControl=sim_en==1

== system npc_controller/IDLE_AND_TIMER/codegen/u32 Data to 2xu16 ==
  u32 Data : Inport
  Bit Shift : hdlsllib/Logic and Bit Operations/Bit Shift  mode=Shift Right Logical  N=8
  Bitwise AND : simulink/Logic and Bit Operations/Bitwise Operator  logicop=AND  UseBitMask=on  BitMask=bin2dec('00000000000000001111111111111111')  BitMaskRealWorld=Stored Integer
  Bitwise AND1 : simulink/Logic and Bit Operations/Bitwise Operator  logicop=AND  UseBitMask=on  BitMask=hex2dec('FFFF0000')  BitMaskRealWorld=Stored Integer
  Data Type Conversion : DataTypeConversion  OutDataTypeStr=uint16  SaturateOnIntegerOverflow=off  RndMeth=Floor
  Data Type Conversion1 : DataTypeConversion  OutDataTypeStr=uint16  SaturateOnIntegerOverflow=off  RndMeth=Floor
  u16Lsb : Outport
  u16Msb : Outport  Port=2
  wires:
  u32 Data/1 -> Bitwise AND1/1, Bitwise AND/1
  Bit Shift/1 -> Data Type Conversion1/1
  Bitwise AND/1 -> Data Type Conversion/1
  Data Type Conversion1/1 -> u16Msb/1
  Bitwise AND1/1 -> Bit Shift/1
  Data Type Conversion/1 -> u16Lsb/1

== system npc_controller/CONTROL/CONTROL/false/CLA_CONTROL ==
  va : Inport  OutDataTypeStr=single
  vb : Inport  Port=2  OutDataTypeStr=single
  vc : Inport  Port=3  OutDataTypeStr=single
  ia : Inport  Port=4  OutDataTypeStr=single
  ib : Inport  Port=5  OutDataTypeStr=single
  ic : Inport  Port=6  OutDataTypeStr=single
  vbulk : Inport  Port=7  OutDataTypeStr=single
  vmid : Inport  Port=8  OutDataTypeStr=single
  control_en : Inport  Port=9
  ref : Inport  Port=10
  angle : Inport  Port=11
  pol_pha : Inport  Port=12
  pol_phb : Inport  Port=13
  pol_phc : Inport  Port=14
  pha_en1 : Inport  Port=15
  phb_en1 : Inport  Port=16
  phc_en1 : Inport  Port=17
  pfc_ok2 : Inport  Port=18  OutDataTypeStr=boolean
  Trigger : TriggerPort  TriggerType=function-call  VariantControl=Variant  PortDimensions=1
  CONTROL : Subsystem
      settings: RTWSystemCode=Inline
  Function-Call Generator : simulink/Ports & Subsystems/Function-Call Generator  sample_time=-1  numberOfIterations=1  DisallowWideOutput=off
  Function-Call Split1 : FunctionCallSplit  NumOutputPorts=2
  Function-Call Split2 : FunctionCallSplit  NumOutputPorts=2
  Function-Call Split3 : FunctionCallSplit  NumOutputPorts=2
  GPIO_HIGH : Subsystem
      settings: RTWSystemCode=Inline
  GPIO_LOW : Subsystem
      settings: RTWSystemCode=Inline
  INIT/RESET_CONTROL : Subsystem
  sim_cmp : Outport
  Vpk : Outport  Port=2
  wires:
  va/1 -> CONTROL/1(adc_out)  "cpu2cla_van"
  vb/1 -> CONTROL/2(adc_out1)  "cpu2cla_vbn"
  vc/1 -> CONTROL/3(adc_out2)  "cpu2cla_vcn"
  ia/1 -> CONTROL/4(adc_out3)  "cpu2cla_ia"
  ib/1 -> CONTROL/5(adc_out4)  "cpu2cla_ib"
  ic/1 -> CONTROL/6(adc_out5)  "cpu2cla_ic"
  vbulk/1 -> CONTROL/7(adc_out6)  "cpu2cla_vbulk"
  vmid/1 -> CONTROL/8(adc_out7)  "cpu2cla_vmid"
  ref/1 -> CONTROL/9(ref)  "cpu2cla_ref"
  Function-Call Split1/2 -> Function-Call Split3/1
  Function-Call Generator/1 -> Function-Call Split1/1
  Function-Call Split2/1 -> CONTROL/Trigger
  Function-Call Split2/2 -> GPIO_LOW/Trigger
  Function-Call Split1/1 -> GPIO_HIGH/Trigger
  CONTROL/1(sim_cmp) -> sim_cmp/1
  control_en/1 -> INIT/RESET_CONTROL/1(control_en)  "cpu2cla_control_en"
  Function-Call Split3/2 -> Function-Call Split2/1
  Function-Call Split3/1 -> INIT/RESET_CONTROL/Trigger
  pol_pha/1 -> CONTROL/11(pol_pha)  "cpu2cla_pol_pha"
  pol_phb/1 -> CONTROL/12(pol_phb)  "cpu2cla_pol_phb"
  pol_phc/1 -> CONTROL/13(pol_phc)  "cpu2cla_pol_phc"
  angle/1 -> CONTROL/10(angle)  "cpu2cla_angle"
  pha_en1/1 -> INIT/RESET_CONTROL/2(pha_en1)  "cpu2cla_pha_en"
  phb_en1/1 -> INIT/RESET_CONTROL/3(phb_en1)  "cpu2cla_phb_en"
  phc_en1/1 -> INIT/RESET_CONTROL/4(phc_en1)  "cpu2cla_phc_en"
  CONTROL/3(Vpk) -> Vpk/1  "cpu2cla_Vpk"
  pfc_ok2/1 -> CONTROL/14(pfc_ok2)  "cpu2cla_pfc_ok2"

== system npc_controller/CONTROL/GET_ADC/ADC/codegen ==
  note: AC_OK - 45 - 60Vrms
  note: Note:
      | A0 VCSB_AD J3.30
      | A1 T_MUX_AD J7.70
      | A2 ICSC_AD J3.29
      | A3 VSCC_AD J3.26
      | A4 ICSA_AD J7.69
      | A5 VCSA_AD J7.66
      |
      | 14 ICSB_AD J3.23
      | 15 VBIAS_AD J7.63
      |
      | B0 IPHASE_A_ADC XX
      | B1 ADC_DEBUG_1 XX
      | B2 IPHASE_B_ADC J3.28
      | B3 IPHASE_C_ADC J3.25
      | B4 VPFC_OUT_AD J7.68
      | B5 VPFC_MID_AD J7.65
      |
      | *Near grid is ics
  adc_in : Inport
  ADCA : Subsystem
  ADCC : Subsystem
  Bus Creator1 : BusCreator  Inputs=8  OutDataTypeStr=Bus: adc
  Bus Creator2 : BusCreator  Inputs=8  OutDataTypeStr=Bus: adc_rect
  Data Store Read : DataStoreRead  Commented=on  DataStoreName=adc_vbulk  IndexOptions=Index vector (dialog)  Indices=1  OutputSizes=1
  Data Store Read1 : DataStoreRead  Commented=on  DataStoreName=adc_vmid  IndexOptions=Index vector (dialog)  Indices=1  OutputSizes=1
  Data Store Read2 : DataStoreRead  Commented=on  DataStoreName=rms_va  IndexOptions=Index vector (dialog)  Indices=1  OutputSizes=1
  Data Store Read3 : DataStoreRead  Commented=on  DataStoreName=rms_vb  IndexOptions=Index vector (dialog)  Indices=1  OutputSizes=1
  Data Store Read4 : DataStoreRead  Commented=on  DataStoreName=rms_vc  IndexOptions=Index vector (dialog)  Indices=1  OutputSizes=1
  Data Store Write : DataStoreWrite  Commented=on  DataStoreName=ac_ok  IndexOptions=Index vector (dialog)  Indices=1  OutputSizes=1
  Data Store Write7 : DataStoreWrite  Commented=on  DataStoreName=adc_vtop  IndexOptions=Index vector (dialog)  Indices=1  OutputSizes=1
  Function-Call Generator : simulink/Ports & Subsystems/Function-Call Generator  sample_time=-1  numberOfIterations=1  DisallowWideOutput=off
  Function-Call Split2 : FunctionCallSplit  NumOutputPorts=2
  IIR Filter7 : Subsystem  Commented=on
  If : If  Commented=on  NumInputs=3  IfExpression=u1 < 100 & u2 < 100 & u3 < 100
  If Action Subsystem : Subsystem  Commented=on  TreatAsAtomicUnit=on
  If Action Subsystem1 : Subsystem  Commented=on  TreatAsAtomicUnit=on
  If Action Subsystem2 : Subsystem  Commented=on  TreatAsAtomicUnit=on
  If Action Subsystem3 : Subsystem  Commented=on  TreatAsAtomicUnit=on
  If1 : If  Commented=on  NumInputs=3  IfExpression=u1 > 134 & u2 > 134 & u3 > 134
  Merge : Merge  Commented=on  Inputs=4
  Subsystem : Subsystem
  Subsystem1 : Subsystem
  Subsystem2 : Subsystem
  Subsystem3 : Subsystem
  Subsystem4 : Subsystem
  Subsystem5 : Subsystem
  Subsystem6 : Subsystem
  Subsystem7 : Subsystem
  Subsystem8 : Subsystem
  Subtract : Sum  Commented=on  Inputs=+-
  adc_out : Outport
  adc_rect : Outport  Port=2
  wires:
  Data Store Read/1 -> Subtract/1
  Data Store Read1/1 -> Subtract/2
  Subtract/1 -> Data Store Write7/1
  [ic] -> Bus Creator1/6  "ic"
  [va] -> Bus Creator1/1  "va"
  [vb] -> Bus Creator1/2  "vb"
  [vc] -> Bus Creator1/3  "vc"
  [vmid] -> Bus Creator1/8  "vmid"
  [vbulk] -> Bus Creator1/7  "vbulk"
  Bus Creator1/1 -> adc_out/1  "vbulk"
  [ib] -> Bus Creator1/5  "ib"
  [ia] -> Bus Creator1/4  "ia"
  [ia] -> Subsystem3/1(adc)  "ia"
  [va] -> Subsystem/1(adc)  "va"
  Subsystem/1(adc_rect) -> Bus Creator2/1  "va"
  [ic] -> Subsystem5/1(adc)  "ic"
  [vb] -> Subsystem1/1(adc)  "vb"
  [vmid] -> Bus Creator2/8  "vmid"
  [vc] -> Subsystem2/1(adc)  "vc"
  Subsystem5/1(adc_rect) -> Bus Creator2/6  "ic"
  [ib] -> Subsystem4/1(adc)  "ib"
  Subsystem2/1(adc_rect) -> Bus Creator2/3  "vc"
  Subsystem4/1(adc_rect) -> Bus Creator2/5  "ib"
  Subsystem3/1(adc_rect) -> Bus Creator2/4  "ia"
  Subsystem1/1(adc_rect) -> Bus Creator2/2  "vb"
  [vbulk] -> Bus Creator2/7  "vbulk"
  Bus Creator2/1 -> adc_rect/1
  Function-Call Split2/1 -> ADCA/Trigger
  Function-Call Generator/1 -> Function-Call Split2/1
  ADCA/1(vb) -> [vb]
  ADCA/4(ia) -> [ia]
  ADCA/3(vc) -> [vc]
  ADCA/2(ic) -> [ic]
  ADCA/5(va) -> [va]
  ADCA/6(ib) -> [ib]
  ADCC/4(vbulk) -> [vbulk]
  ADCC/5(vmid) -> [vmid]
  Function-Call Split2/2 -> ADCC/Trigger
  ADCC/3(iphasec) -> [iphasec]
  ADCC/2(iphaseb) -> [iphaseb]
  ADCC/1(iphasea) -> [iphasea]
  [iphasec] -> Subsystem8/1(adc)  "vc"
  [iphaseb] -> Subsystem7/1(adc)  "vb"
  [iphasea] -> Subsystem6/1(adc)  "va"
  Data Store Read3/1 -> If1/2, If/2
  Data Store Read4/1 -> If1/3, If/3
  Data Store Read2/1 -> If1/1, If/1
  If/1 -> If Action Subsystem/Action
  If1/1 -> If Action Subsystem1/Action
  If Action Subsystem/1(Out1) -> Merge/1
  If/2 -> If Action Subsystem2/Action
  If Action Subsystem2/1(Out1) -> Merge/2
  If Action Subsystem1/1(Out1) -> Merge/3
  If1/2 -> If Action Subsystem3/Action
  If Action Subsystem3/1(Out1) -> Merge/4
  Merge/1 -> Data Store Write/1

== system npc_controller/CONTROL/GET_ADC/ADC/sim ==
  note: Notes:
      | vac_adc = vac_actual*0.00264706+1.65
      | iac_adc = iac_actual*0.02+1.65
      | vbulk_adc = vbulk_actual*3.49e-3
      | vmid_adc = vmid_acutal*3.49e-3
  note: Note:
      | Vmid         C2
      | Vbulk        A5
      |
      | Va            A2/B6
      | Vb            B0
      | Vc            C0
      |
      | Ia             A3
      | Ib             A10/B1, C10
      | Ic             C1
  note: since the current sense in hardware is -ve
  adc_in : Inport
  Bus Creator1 : BusCreator  Inputs=8  OutDataTypeStr=Bus: adc
  Bus Creator2 : BusCreator  Inputs=8  OutDataTypeStr=Bus: adc_rect
  Cast To Single : DataTypeConversion  OutDataTypeStr=single  SaturateOnIntegerOverflow=off  RndMeth=Floor
  Cast To Single1 : DataTypeConversion  OutDataTypeStr=single  SaturateOnIntegerOverflow=off  RndMeth=Floor
  Data Store Read : DataStoreRead  DataStoreName=adc_offset_vc  IndexOptions=Index vector (dialog)  Indices=1  OutputSizes=1
  Data Store Read1 : DataStoreRead  DataStoreName=adc_offset_ic  IndexOptions=Index vector (dialog)  Indices=1  OutputSizes=1
  Data Store Read2 : DataStoreRead  DataStoreName=adc_offset_vb  IndexOptions=Index vector (dialog)  Indices=1  OutputSizes=1
  Data Store Read4 : DataStoreRead  DataStoreName=adc_offset_va  IndexOptions=Index vector (dialog)  Indices=1  OutputSizes=1
  Data Store Read6 : DataStoreRead  DataStoreName=adc_offset_ia  IndexOptions=Index vector (dialog)  Indices=1  OutputSizes=1
  Data Store Read7 : DataStoreRead  DataStoreName=adc_offset_ib  IndexOptions=Index vector (dialog)  Indices=1  OutputSizes=1
  Demux : Demux  Outputs=8
  Gain : Gain  Gain=1.41  ParamDataTypeStr=single  OutDataTypeStr=single
  IIR Filter1 : Subsystem
  IIR Filter3 : Subsystem
  IIR Filter5 : Subsystem  Commented=on
  IIR Filter8 : Subsystem
  Scope : Scope  NumInputPorts=2
  Scope1 : Scope  NumInputPorts=2
  Scope2 : Scope
  Scope3 : Scope
  Scope4 : Scope  NumInputPorts=3
  Subsystem : Subsystem
  Subsystem1 : Subsystem
  Subsystem2 : Subsystem
  Subsystem3 : Subsystem
  Subsystem4 : Subsystem
  Subsystem5 : Subsystem
  vabc{1..6} (6 alike) : Sum  Inputs=|+-  AccumDataTypeStr=single  OutDataTypeStr=single
  adc_out : Outport
  adc_rect : Outport  Port=2
  wires:
  adc_in/1 -> Demux/1
  Demux/7 -> Cast To Single/1
  Cast To Single/1 -> IIR Filter3/1(x[n])
  Data Store Read6/1 -> vabc2/2
  Demux/4 -> vabc2/1
  vabc2/1 -> [ia]
  Bus Creator1/1 -> adc_out/1  "vbulk"
  Demux/6 -> vabc6/1
  Data Store Read2/1 -> vabc1/2
  Data Store Read1/1 -> Scope3/1, vabc6/2
  Data Store Read7/1 -> vabc5/2
  Demux/5 -> vabc5/1
  Demux/2 -> vabc1/1
  vabc3/1 -> [va]
  Data Store Read/1 -> Scope2/1, vabc4/2
  Data Store Read4/1 -> vabc3/2
  vabc1/1 -> [vb]
  Cast To Single1/1 -> IIR Filter8/1(x[n])
  vabc5/1 -> [ib]
  Demux/3 -> vabc4/1
  Demux/1 -> vabc3/1  "va"
  Demux/8 -> Cast To Single1/1  "vmid"
  [vb] -> Bus Creator1/2  "vb"
  [vc] -> Bus Creator1/3  "vc"
  [ia] -> Bus Creator1/4  "ia"
  [ib] -> Bus Creator1/5  "ib"
  [ic] -> Bus Creator1/6  "ic"
  [va] -> Bus Creator1/1  "va"
  [vbulk] -> Bus Creator1/7  "vbulk"
  [vmid] -> Bus Creator1/8  "vmid"
  Subsystem/1(adc_rect) -> Scope4/1, IIR Filter1/1(x[n]), Scope/2, Bus Creator2/1  "va"
  Subsystem1/1(adc_rect) -> Bus Creator2/2  "vb"
  Subsystem3/1(adc_rect) -> Scope1/2, Bus Creator2/4  "ia"
  Subsystem4/1(adc_rect) -> Bus Creator2/5  "ib"
  Bus Creator2/1 -> adc_rect/1  "vbulk"
  [va] -> Subsystem/1(adc), Scope/1  "va"
  [vb] -> Subsystem1/1(adc)  "vb"
  [vc] -> Subsystem2/1(adc)  "vc"
  [ia] -> Scope1/1, Subsystem3/1(adc)  "ia"
  [ib] -> Subsystem4/1(adc)  "ib"
  [ic] -> Subsystem5/1(adc)  "ic"
  [vmid] -> Bus Creator2/8  "vmid"
  [vbulk] -> Bus Creator2/7  "vbulk"
  Subsystem2/1(adc_rect) -> Bus Creator2/3  "vc"
  Subsystem5/1(adc_rect) -> Bus Creator2/6  "ic"
  vabc4/1 -> [vc]  "va"
  vabc6/1 -> [ic]  "va"
  IIR Filter3/1(y[n]) -> [vbulk]
  IIR Filter8/1(y[n]) -> [vmid]
  IIR Filter1/1(y[n]) -> Scope4/2, Gain/1  "va"
  Gain/1 -> Scope4/3

== system npc_controller/CONTROL/POLARITY/PLL_Block1/SRF_PLL ==
  Vabc : Inport
  Demux1 : Demux  Outputs=3
  Gain : Gain  Commented=on  Gain=1/(2*pi)
  Integrator : Subsystem
  Memory : Memory  InheritSampleTime=on  LinearizeAsDelay=on
  PI : Subsystem
  Subsystem1 : Subsystem  Commented=on
  Sum1 : Sum  Inputs=|++  AccumDataTypeStr=single  OutDataTypeStr=single
  abc to dq : Subsystem
  f0 : Constant  Value=2*pi*50  OutDataTypeStr=fixdt('single', 'DataTypeOverride', 'Off')
  SinVal : Outport  VectorParamsAs1DForOutWhenUnconnected=off
  CosVal : Outport  Port=2  VectorParamsAs1DForOutWhenUnconnected=off
  theta : Outport  Port=3  OutDataTypeStr=single  VectorParamsAs1DForOutWhenUnconnected=off
  wires:
  Vabc/1 -> Demux1/1
  Memory/1 -> abc to dq/4(wt)
  Integrator/1(wt) -> Memory/1, theta/1
  abc to dq/1(q) -> PI/1(Vq)
  f0/1 -> Sum1/2
  Gain/1 -> Subsystem1/1(x[n])  "Freq_Unf"
  PI/1(PI Out) -> Sum1/1
  Sum1/1 -> Gain/1, Integrator/1(PI Out)
  Demux1/1 -> abc to dq/1(a)
  Demux1/2 -> abc to dq/2(b)
  Demux1/3 -> abc to dq/3(c)

== system npc_controller/CONTROL/POLARITY/PLL_Block1/Subsystem ==
  In1 : Inport
  Cast To Single : DataTypeConversion  OutDataTypeStr=single  SaturateOnIntegerOverflow=off  RndMeth=Floor
  Constant2 : Constant  Value=0
  GreaterThan1 : RelationalOperator  Operator=>  OutDataTypeStr=boolean  RndMeth=Simplest  InputSameDT=off
  Initialize at Zero Crossing : Subsystem  TreatAsAtomicUnit=on
  Out1 : Outport
  wires:
  GreaterThan1/1 -> Initialize at Zero Crossing/Trigger, Initialize at Zero Crossing/1(In1)
  Constant2/1 -> GreaterThan1/2
  Initialize at Zero Crossing/1(Out1) -> Cast To Single/1
  In1/1 -> GreaterThan1/1
  Cast To Single/1 -> Out1/1

== system npc_controller/CONTROL/STATE-MACHINE/CPU_CONTROL_100_A2_precharge_pfc_ok2/configFutDis/System Outputs1 ==

== system npc_controller/CONTROL/STATE-MACHINE/CPU_CONTROL_100_A2_precharge_pfc_ok2/configFutDis/System Outputs2 ==

== system npc_controller/CONTROL/STATE-MACHINE/CPU_CONTROL_100_A2_precharge_pfc_ok2/configFutEn/System Outputs1 ==
